simulink model "SVPWM_mdl"  (Simulink 9.0)
settings: Solver=VariableStepAuto  StartTime=0.0  StopTime=10.0  RelTol=1e-3
libraries: simulink x4
settings Model: Creator=80573  LastModifiedBy=80573
settings DataIOCC: SaveFormat=Dataset
settings OptimizationCC: LifeSpan=auto
settings DebuggingCC: UnderspecifiedInitializationDetection=Simplified  MergeDetectMultiDrivingBlocksExec=error  SFUnexpectedBacktrackingDiag=error  SFNoUnconditionalDefaultTransitionDiag=error  SFExecutionAtInitializationDiag=warning
settings HardwareCC: ProdBitPerPointer=64  ProdBitPerSizeT=64  ProdBitPerPtrDiffT=64  ProdLargestAtomicFloat=Float  ProdIntDivRoundTo=Zero  ProdEndianess=LittleEndian  ProdWordSize=64  ProdHWDeviceType=Intel->x86-64 (Windows64)
settings ModelReferenceCC: PropagateSignalLabelsOutOfModel=on
settings CodeAppCC: StateflowObjectComments=off
settings GRTTargetCC: TargetLangStandard=C99 (ISO)
settings ConfigComp: CovMetricSettings=dwe  CovHtmlReporting=off  CovSaveCumulativeToWorkspaceVar=off  CovSaveSingleToWorkspaceVar=off  CovExternalEMLEnable=on

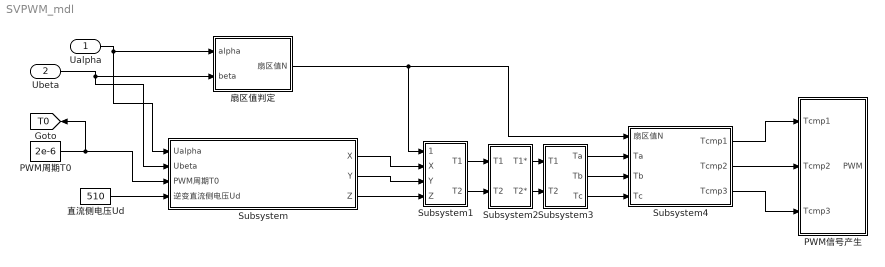
== system SVPWM_mdl ==
  Ualpha : Inport
  Ubeta : Inport  Port=2
  PWM信号产生 : Subsystem
  PWM周期T0 : Constant  Value=2e-6
  Subsystem : Subsystem
  Subsystem1 : Subsystem
  Subsystem2 : Subsystem
  Subsystem3 : Subsystem
  Subsystem4 : Subsystem
  扇区值判定 : Subsystem
  直流侧电压Ud : Constant  Value=510
  tag scope: T0=global
  wires:
  Subsystem1/1(T1) -> Subsystem2/1(T1)
  Subsystem1/2(T2) -> Subsystem2/2(T2)
  Subsystem2/1(T1*) -> Subsystem3/1(T1)
  Subsystem2/2(T2*) -> Subsystem3/2(T2)
  Subsystem3/1(Ta) -> Subsystem4/2(Ta)
  Subsystem3/2(Tb) -> Subsystem4/3(Tb)
  Subsystem3/3(Tc) -> Subsystem4/4(Tc)
  Subsystem4/1(Tcmp1) -> PWM信号产生/1(Tcmp1)
  Subsystem4/2(Tcmp2) -> PWM信号产生/2(Tcmp2)
  Subsystem4/3(Tcmp3) -> PWM信号产生/3(Tcmp3)
  Subsystem/1(X) -> Subsystem1/2(X)
  Subsystem/2(Y) -> Subsystem1/3(Y)
  Subsystem/3(Z) -> Subsystem1/4(Z)
  扇区值判定/1(扇区值N) -> Subsystem1/1(扇区值N), Subsystem4/1(扇区值N)
  Ubeta/1 -> Subsystem/2(Ubeta), 扇区值判定/2(beta)
  PWM周期T0/1 -> Subsystem/3(PWM周期T0), [T0]
  Ualpha/1 -> Subsystem/1(Ualpha), 扇区值判定/1(alpha)
  直流侧电压Ud/1 -> Subsystem/4(逆变直流侧电压Ud)

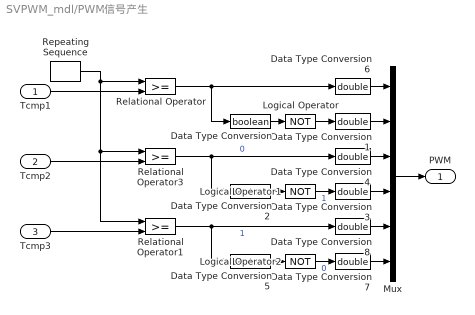
== system SVPWM_mdl/PWM信号产生 ==
  Tcmp1 : Inport
  Tcmp2 : Inport  Port=2
  Tcmp3 : Inport  Port=3
  Data Type Conversion : DataTypeConversion  OutDataTypeStr=boolean
  Data Type Conversion{1,3..4,6..8} (6 alike) : DataTypeConversion  OutDataTypeStr=double
  Data Type Conversion2 : DataTypeConversion  OutDataTypeStr=boolean
  Data Type Conversion5 : DataTypeConversion  OutDataTypeStr=boolean
  Logical Operator : Logic  Operator=NOT  AllPortsSameDT=off  OutDataTypeStr=boolean
  Logical Operator1 : Logic  Operator=NOT  AllPortsSameDT=off  OutDataTypeStr=boolean
  Logical Operator2 : Logic  Operator=NOT  AllPortsSameDT=off  OutDataTypeStr=boolean
  Mux : Mux  Inputs=6
  Relational Operator : RelationalOperator  OutDataTypeStr=boolean  RndMeth=Nearest
  Relational Operator1 : RelationalOperator  OutDataTypeStr=boolean  RndMeth=Nearest
  Relational Operator3 : RelationalOperator  OutDataTypeStr=boolean  RndMeth=Nearest
  Repeating Sequence : simulink/Sources/Repeating Sequence  rep_seq_t=[0 1e-4 2e-4]  rep_seq_y=[0 1.3e-6 0]
  PWM : Outport
  wires:
  Data Type Conversion/1 -> Logical Operator/1
  Logical Operator/1 -> Data Type Conversion1/1
  Relational Operator/1 -> Data Type Conversion6/1, Data Type Conversion/1
  Logical Operator1/1 -> Data Type Conversion3/1  "1"
  Relational Operator3/1 -> Data Type Conversion4/1, Data Type Conversion2/1  "0"
  Data Type Conversion2/1 -> Logical Operator1/1
  Relational Operator1/1 -> Data Type Conversion8/1, Data Type Conversion5/1  "1"
  Data Type Conversion5/1 -> Logical Operator2/1
  Logical Operator2/1 -> Data Type Conversion7/1  "0"
  Repeating Sequence/1 -> Relational Operator1/1, Relational Operator3/1, Relational Operator/1
  Tcmp1/1 -> Relational Operator/2
  Tcmp2/1 -> Relational Operator3/2
  Tcmp3/1 -> Relational Operator1/2
  Data Type Conversion6/1 -> Mux/1
  Data Type Conversion1/1 -> Mux/2
  Data Type Conversion4/1 -> Mux/3
  Data Type Conversion3/1 -> Mux/4
  Data Type Conversion8/1 -> Mux/5
  Data Type Conversion7/1 -> Mux/6
  Mux/1 -> PWM/1

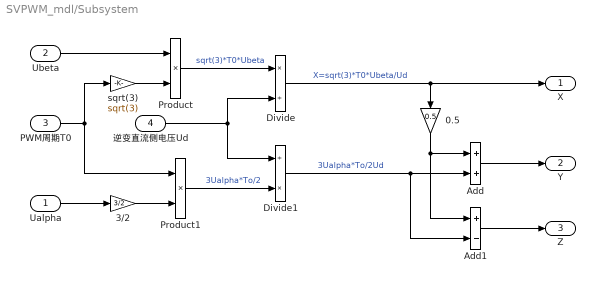
== system SVPWM_mdl/Subsystem ==
  Ualpha : Inport
  Ubeta : Inport  Port=2
  PWM周期T0 : Inport  Port=3
  逆变直流侧电压Ud : Inport  Port=4
  0.5 : Gain  Gain=0.5
  3/2 : Gain  Gain=3/2
  Add : Sum
  Add1 : Sum  Inputs=+-
  Divide : Product  Inputs=*/
  Divide1 : Product  Inputs=/*
  Product : Product
  Product1 : Product
  "sqrt(3) " : Gain  Gain=sqrt(3)
  X : Outport
  Y : Outport  Port=2
  Z : Outport  Port=3
  wires:
  Divide/1 -> X/1, 0.5/1  "X=sqrt(3)*T0*Ubeta/Ud"
  逆变直流侧电压Ud/1 -> Divide1/1, Divide/2
  0.5/1 -> Add/1, Add1/1
  PWM周期T0/1 -> "sqrt(3) "/1, Product1/1
  "sqrt(3) "/1 -> Product/2
  3/2/1 -> Product1/2
  Product1/1 -> Divide1/2  "3Ualpha*To/2"
  Add/1 -> Y/1
  Ualpha/1 -> 3/2/1
  Ubeta/1 -> Product/1
  Divide1/1 -> Add1/2, Add/2  "3Ualpha*To/2Ud"
  Add1/1 -> Z/1
  Product/1 -> Divide/1  "sqrt(3)*T0*Ubeta"

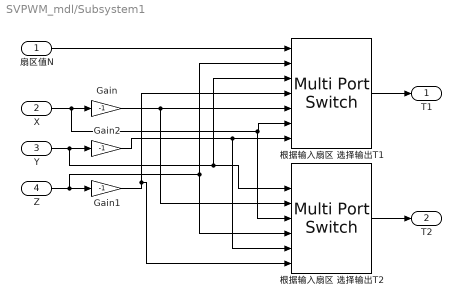
== system SVPWM_mdl/Subsystem1 ==
  扇区值N : Inport
  X : Inport  Port=2
  Y : Inport  Port=3
  Z : Inport  Port=4
  Gain : Gain  Gain=-1
  Gain1 : Gain  Gain=-1
  Gain2 : Gain  Gain=-1
  根据输入扇区 选择输出T1 : MultiPortSwitch  Inputs=6
  根据输入扇区 选择输出T2 : MultiPortSwitch  Inputs=6
  T1 : Outport
  T2 : Outport  Port=2
  wires:
  X/1 -> 根据输入扇区 选择输出T2/4, 根据输入扇区 选择输出T1/6, Gain/1
  Y/1 -> 根据输入扇区 选择输出T1/3, 根据输入扇区 选择输出T2/2, Gain2/1
  Z/1 -> 根据输入扇区 选择输出T2/5, 根据输入扇区 选择输出T1/2, Gain1/1
  Gain1/1 -> 根据输入扇区 选择输出T2/7, 根据输入扇区 选择输出T1/4
  Gain/1 -> 根据输入扇区 选择输出T1/5, 根据输入扇区 选择输出T2/3
  根据输入扇区 选择输出T1/1 -> T1/1
  根据输入扇区 选择输出T2/1 -> T2/1
  Gain2/1 -> 根据输入扇区 选择输出T2/6, 根据输入扇区 选择输出T1/7
  扇区值N/1 -> 根据输入扇区 选择输出T1/1

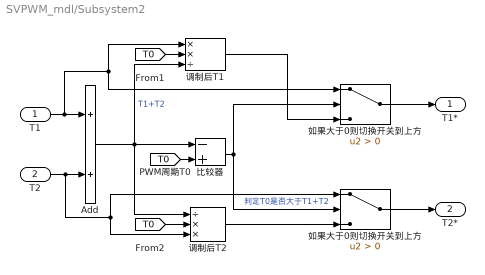
== system SVPWM_mdl/Subsystem2 ==
  T1 : Inport
  T2 : Inport  Port=2
  Add : Sum
  如果大于0则切换开关到上方 : Switch  Criteria=u2 > Threshold
  "如果大于0则切换开关到上方 " : Switch  Criteria=u2 > Threshold
  比较器 : Sum  Inputs=-+
  调制后T1 : Product  Inputs=**/
  调制后T2 : Product  Inputs=/**
  T1* : Outport
  T2* : Outport  Port=2
  wires:
  调制后T1/1 -> 如果大于0则切换开关到上方/3
  "如果大于0则切换开关到上方 "/1 -> T2*/1
  比较器/1 -> "如果大于0则切换开关到上方 "/2, 如果大于0则切换开关到上方/2  "判定T0是否大于T1+T2"
  [T0] -> 调制后T2/2
  Add/1 -> 调制后T2/1, 比较器/1, 调制后T1/3  "T1+T2"
  [T0] -> 调制后T1/2
  T1/1 -> 如果大于0则切换开关到上方/1, 调制后T1/1, Add/1
  [T0] -> 比较器/2
  如果大于0则切换开关到上方/1 -> T1*/1
  调制后T2/1 -> "如果大于0则切换开关到上方 "/3
  T2/1 -> "如果大于0则切换开关到上方 "/1, 调制后T2/3, Add/2

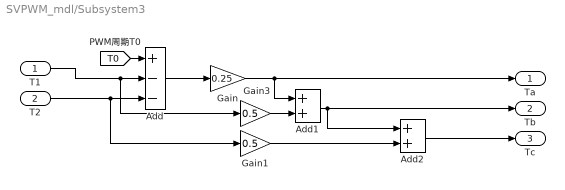
== system SVPWM_mdl/Subsystem3 ==
  T1 : Inport
  T2 : Inport  Port=2
  Add : Sum  Inputs=+--
  Add1 : Sum
  Add2 : Sum
  Gain : Gain  Gain=0.25
  Gain1 : Gain  Gain=0.5
  Gain3 : Gain  Gain=0.5
  Ta : Outport
  Tb : Outport  Port=2
  Tc : Outport  Port=3
  wires:
  Add2/1 -> Tc/1
  Add/1 -> Gain/1
  [T0] -> Add/1
  T1/1 -> Gain3/1, Add/2
  Add1/1 -> Tb/1, Add2/1
  Gain3/1 -> Add1/2
  Gain1/1 -> Add2/2
  Gain/1 -> Ta/1, Add1/1
  T2/1 -> Gain1/1, Add/3

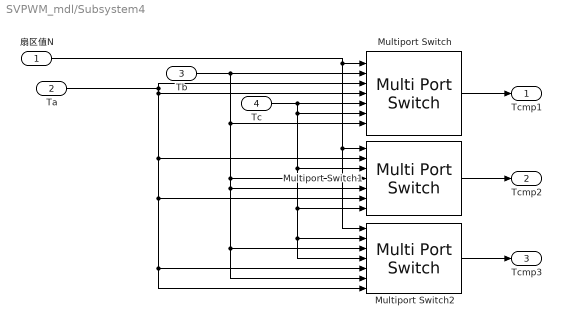
== system SVPWM_mdl/Subsystem4 ==
  扇区值N : Inport
  Ta : Inport  Port=2
  Tb : Inport  Port=3
  Tc : Inport  Port=4
  Multiport Switch : MultiPortSwitch  Inputs=6  OutDataTypeStr=double
  Multiport Switch1 : MultiPortSwitch  Inputs=6  OutDataTypeStr=double
  Multiport Switch2 : MultiPortSwitch  Inputs=6  OutDataTypeStr=double
  Tcmp1 : Outport
  Tcmp2 : Outport  Port=2
  Tcmp3 : Outport  Port=3
  wires:
  扇区值N/1 -> Multiport Switch2/1, Multiport Switch1/1, Multiport Switch/1
  Tb/1 -> Multiport Switch2/6, Multiport Switch2/3, Multiport Switch1/5, Multiport Switch1/4, Multiport Switch/7, Multiport Switch/2
  Multiport Switch/1 -> Tcmp1/1
  Ta/1 -> Multiport Switch/3, Multiport Switch/4, Multiport Switch2/7, Multiport Switch2/5, Multiport Switch1/6, Multiport Switch1/2
  Multiport Switch1/1 -> Tcmp2/1
  Tc/1 -> Multiport Switch1/7, Multiport Switch2/2, Multiport Switch2/4, Multiport Switch1/3, Multiport Switch/6, Multiport Switch/5
  Multiport Switch2/1 -> Tcmp3/1

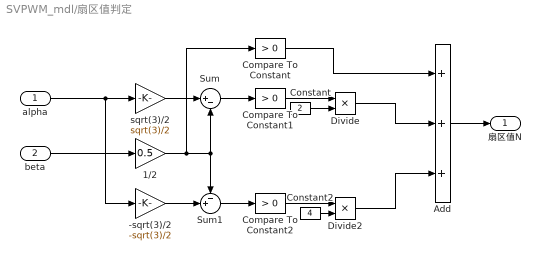
== system SVPWM_mdl/扇区值判定 ==
  alpha : Inport
  beta : Inport  Port=2
  -sqrt(3)/2 : Gain  Gain=-sqrt(3)/2
  1/2 : Gain  Gain=0.5
  "Add " : Sum  Inputs=+++
  Compare To Constant : simulink/Logic and Bit Operations/Compare To Constant  relop=>  const=0  OutDataTypeStr=boolean
  Compare To Constant1 : simulink/Logic and Bit Operations/Compare To Constant  relop=>  const=0  OutDataTypeStr=boolean
  Compare To Constant2 : simulink/Logic and Bit Operations/Compare To Constant  relop=>  const=0  OutDataTypeStr=boolean
  Constant : Constant  Value=2
  Constant2 : Constant  Value=4
  Divide : Product  Inputs=**
  Divide2 : Product  Inputs=**
  Sum : Sum  Inputs=|+-
  Sum1 : Sum  Inputs=-+|
  sqrt(3)/2 : Gain  Gain=sqrt(3)/2
  扇区值N : Outport
  wires:
  Divide2/1 -> "Add "/3
  Sum/1 -> Compare To Constant1/1
  -sqrt(3)/2/1 -> Sum1/2
  Sum1/1 -> Compare To Constant2/1
  Constant2/1 -> Divide2/2
  1/2/1 -> Sum1/1, Sum/2, Compare To Constant/1
  "Add "/1 -> 扇区值N/1
  Compare To Constant2/1 -> Divide2/1
  beta/1 -> 1/2/1
  sqrt(3)/2/1 -> Sum/1
  Compare To Constant/1 -> "Add "/1
  Compare To Constant1/1 -> Divide/1
  Divide/1 -> "Add "/2
  Constant/1 -> Divide/2
  alpha/1 -> -sqrt(3)/2/1, sqrt(3)/2/1
